simulink model "Quadprog_LF_constraint"  (R2024b)
settings: Solver=FixedStepAuto  StartTime=0.0  StopTime=20  FixedStep=Ts  RelTol=1e-3
model workspace (MAT data in the model file):
  Ts = 0.001
  a = 0.8
settings Model: Creator=sara  LastModifiedBy=Negin Service
settings SolverCC: AlgebraicLoopSolver=TrustRegion
settings RTWCC: GPUComputeCapability=3.5

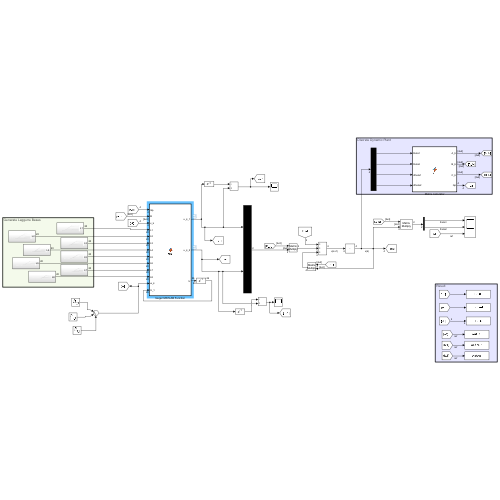
[thumbnail: Simulink's stored preview of the top-level diagram]
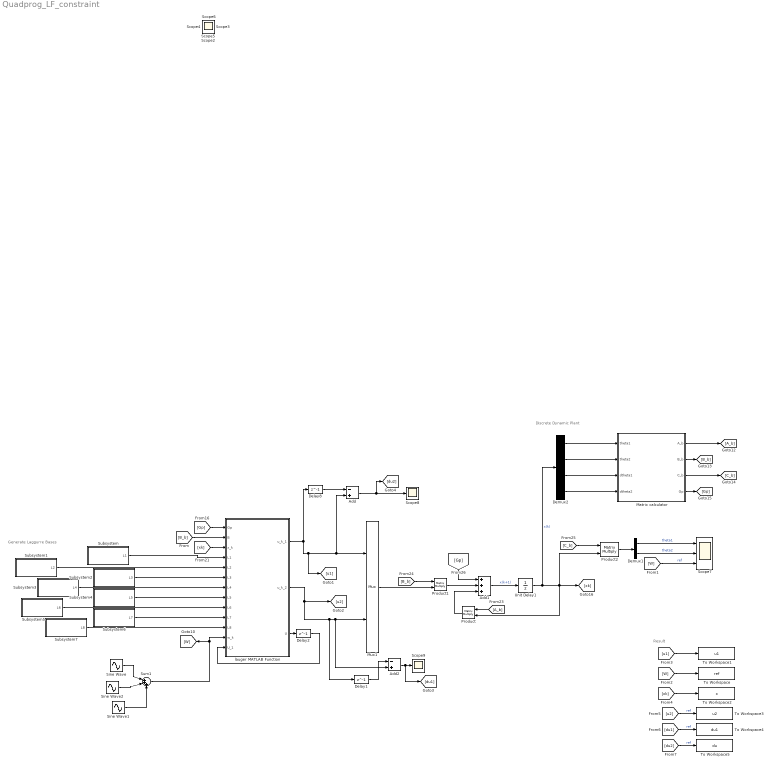
== system Quadprog_LF_constraint ==
  note: Result
  note: Discrete Dynamic Plant
  note: Generate Laggurre Bases
  Add : Sum  Inputs=-+
  Add1 : Sum  Inputs=+++
  Add2 : Sum  Inputs=-+
  Delay1 : Delay  DelayLength=1  SampleTime=Ts
  Delay2 : Delay  DelayLength=1  SampleTime=Ts
  Delay8 : Delay  DelayLength=1  SampleTime=Ts
  Demux1 : Demux  Outputs=2
  Demux2 : Demux
  Matrix calculator : MATLAB Function  TreatAsAtomicUnit=on
  Mux1 : Mux  Inputs=2
  Product : Product  Multiplication=Matrix(*)
  Product1 : Product  Multiplication=Matrix(*)
  Product2 : Product  Multiplication=Matrix(*)
  Scope7 : Scope  NumInputPorts=3
  Scope{,1..6,8..9} (9 alike) : Scope
  Sine Wave : Sin  Amplitude=4  Frequency=0.5  SampleTime=Ts
  Sine Wave1 : Sin  Amplitude=4  SampleTime=Ts
  Sine Wave2 : Sin  Amplitude=4  Frequency=1.5  SampleTime=Ts
  Subsystem : Subsystem
  Subsystem1 : Subsystem
  Subsystem2 : Subsystem
  Subsystem3 : Subsystem
  Subsystem4 : Subsystem
  Subsystem5 : Subsystem
  Subsystem6 : Subsystem
  Subsystem7 : Subsystem
  Sum1 : Sum  Inputs=|+++
  To Workspace : ToWorkspace  VariableName=ref  SaveFormat=Timeseries  SampleTime=-1
  To Workspace1 : ToWorkspace  VariableName=u1  SaveFormat=Timeseries  SampleTime=-1
  To Workspace2 : ToWorkspace  VariableName=x  SaveFormat=Timeseries  SampleTime=-1
  To Workspace3 : ToWorkspace  VariableName=u2  SaveFormat=Timeseries  SampleTime=-1
  To Workspace4 : ToWorkspace  VariableName=du1  SaveFormat=Timeseries  SampleTime=-1
  To Workspace5 : ToWorkspace  VariableName=du  SaveFormat=Timeseries  SampleTime=-1
  Unit Delay1 : UnitDelay  InitialCondition=[0;0;0;0]  SampleTime=Ts  HasFrameUpgradeWarning=on
  lauger MATLAB Function : MATLAB Function  TreatAsAtomicUnit=on
  wires:
  Sine Wave/1 -> Sum1/1
  Subsystem2/1(L3) -> lauger MATLAB Function/6(L3)
  Subsystem/1(L1) -> lauger MATLAB Function/4(L1)
  Subsystem1/1(L2) -> lauger MATLAB Function/5(L2)
  Sum1/1 -> lauger MATLAB Function/12(w_k), [W]
  [B_b] -> lauger MATLAB Function/2(B)
  [xk] -> lauger MATLAB Function/3(x_k)
  [Gp] -> lauger MATLAB Function/1(Gp)
  Mux1/1 -> Product1/2
  Subsystem3/1(L4) -> lauger MATLAB Function/7(L4)
  Subsystem4/1(L5) -> lauger MATLAB Function/8(L5)
  Subsystem5/1(L6) -> lauger MATLAB Function/9(L6)
  Subsystem6/1(L7) -> lauger MATLAB Function/10(L7)
  Subsystem7/1(L8) -> lauger MATLAB Function/11(L8)
  Unit Delay1/1 -> Demux2/1, Product2/2, [xk], Product/2  "x(k)"
  Matrix calculator/1(A_b) -> [A_b]
  Matrix calculator/4(Gp) -> [Gp]
  Matrix calculator/3(C_b) -> [C_b]
  Matrix calculator/2(B_b) -> [B_b]
  [A_b] -> Product/1
  Product/1 -> Add1/3
  [B_b] -> Product1/1
  Product1/1 -> Add1/2
  Add1/1 -> Unit Delay1/1  "x(k+1)"
  [Gp] -> Add1/1
  [C_b] -> Product2/1
  Product2/1 -> Demux1/1
  Demux1/1 -> Scope7/1  "theta1"
  Demux1/2 -> Scope7/2  "theta2"
  Demux2/1 -> Matrix calculator/1(theta1)
  Demux2/2 -> Matrix calculator/2(theta2)
  Demux2/3 -> Matrix calculator/3(dtheta1)
  Demux2/4 -> Matrix calculator/4(dtheta2)
  [W] -> Scope7/3  "ref"
  Sine Wave1/1 -> Sum1/3
  Sine Wave2/1 -> Sum1/2
  Delay8/1 -> Add/1
  Add/1 -> [du2], Scope8/1
  lauger MATLAB Function/1(u_k_1) -> [u1], Add/2, Mux1/1, Delay8/1
  Delay1/1 -> Add2/1
  Add2/1 -> [du1], Scope9/1
  lauger MATLAB Function/2(u_k_2) -> Delay1/1, Add2/2, Mux1/2, [u2]
  [W] -> To Workspace/1
  [u1] -> To Workspace1/1
  [xk] -> To Workspace2/1
  [u2] -> To Workspace3/1  "ref"
  [du1] -> To Workspace4/1  "ref"
  [du2] -> To Workspace5/1  "ref"
  lauger MATLAB Function/3(U) -> Delay2/1
  Delay2/1 -> lauger MATLAB Function/13(U_1)

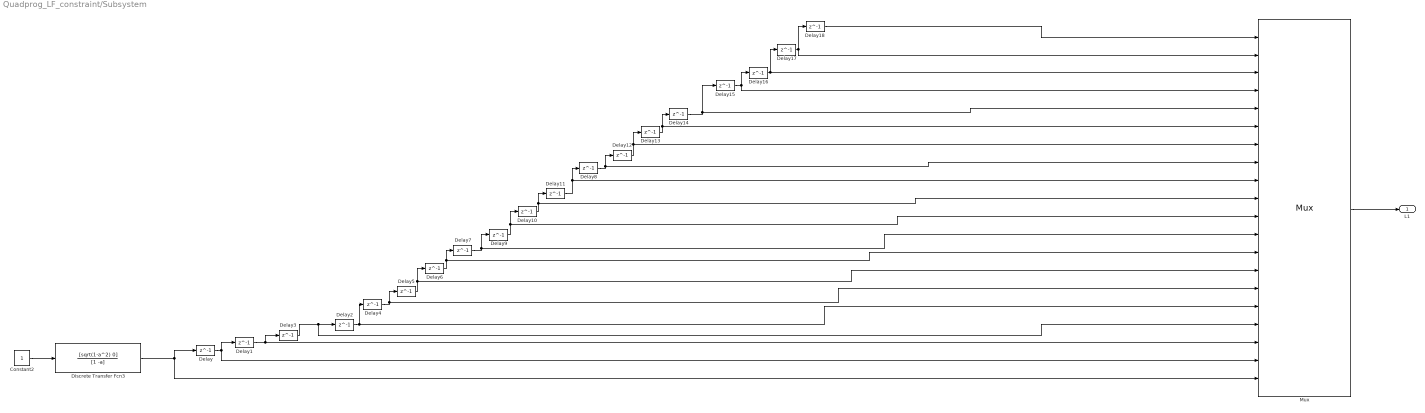
== system Quadprog_LF_constraint/Subsystem ==
  Constant2 : Constant  SampleTime=0.1
  Delay{,1..18} (19 alike) : Delay  DelayLength=1  SampleTime=Ts
  Discrete Transfer Fcn3 : DiscreteTransferFcn  Numerator=[sqrt(1-a^2) 0]  Denominator=[1 -a]  SampleTime=Ts
  Mux : Mux  Inputs=20
  L1 : Outport
  wires:
  Constant2/1 -> Discrete Transfer Fcn3/1
  Delay2/1 -> Mux/16, Delay4/1
  Discrete Transfer Fcn3/1 -> Mux/20, Delay/1
  Delay3/1 -> Mux/17, Delay2/1
  Delay1/1 -> Mux/18, Delay3/1
  Delay/1 -> Mux/19, Delay1/1
  Delay4/1 -> Mux/15, Delay5/1
  Delay5/1 -> Mux/14, Delay6/1
  Delay6/1 -> Mux/13, Delay7/1
  Delay9/1 -> Mux/11, Delay10/1
  Delay7/1 -> Mux/12, Delay9/1
  Delay10/1 -> Mux/10, Delay11/1
  Delay12/1 -> Mux/7, Delay13/1
  Delay8/1 -> Mux/8, Delay12/1
  Delay13/1 -> Delay14/1, Mux/6
  Delay11/1 -> Mux/9, Delay8/1
  Delay16/1 -> Delay17/1, Mux/3
  Delay15/1 -> Delay16/1, Mux/4
  Delay17/1 -> Delay18/1, Mux/2
  Delay14/1 -> Mux/5, Delay15/1
  Mux/1 -> L1/1
  Delay18/1 -> Mux/1

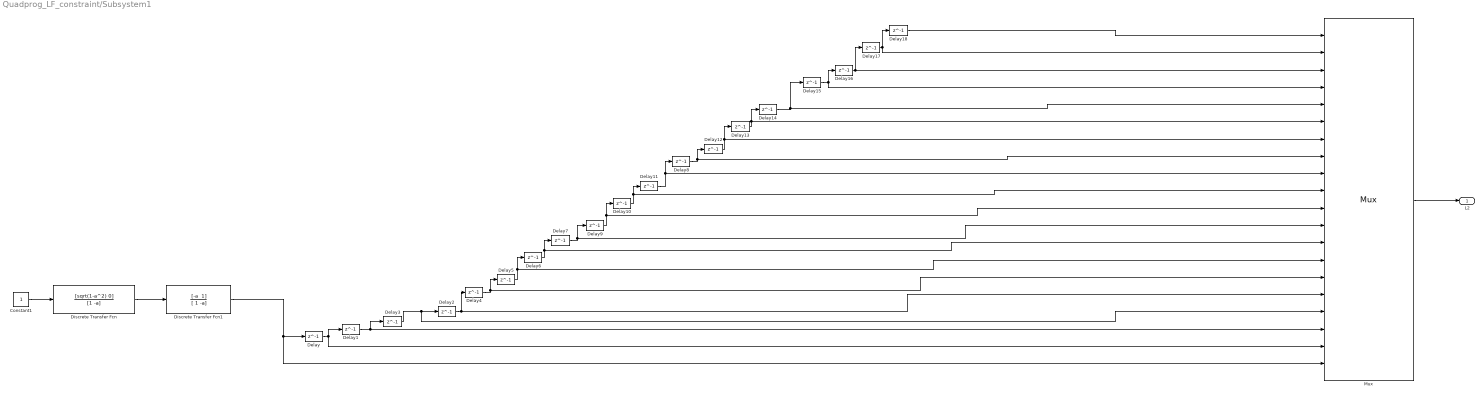
== system Quadprog_LF_constraint/Subsystem1 ==
  Constant1 : Constant  SampleTime=0.1
  Delay{,1..18} (19 alike) : Delay  DelayLength=1  SampleTime=Ts
  Discrete Transfer Fcn : DiscreteTransferFcn  Numerator=[sqrt(1-a^2) 0]  Denominator=[1 -a]  SampleTime=Ts
  Discrete Transfer Fcn1 : DiscreteTransferFcn  Numerator="[-a  1]"  Denominator=[ 1 -a]  SampleTime=Ts
  Mux : Mux  Inputs=20
  L2 : Outport
  wires:
  Delay18/1 -> Mux/1
  Mux/1 -> L2/1
  Delay14/1 -> Delay15/1, Mux/5
  Delay17/1 -> Delay18/1, Mux/2
  Delay15/1 -> Mux/4, Delay16/1
  Delay16/1 -> Mux/3, Delay17/1
  Delay11/1 -> Delay8/1, Mux/9
  Delay13/1 -> Mux/6, Delay14/1
  Delay8/1 -> Delay12/1, Mux/8
  Delay12/1 -> Delay13/1, Mux/7
  Delay10/1 -> Delay11/1, Mux/10
  Delay7/1 -> Delay9/1, Mux/12
  Delay9/1 -> Delay10/1, Mux/11
  Delay6/1 -> Delay7/1, Mux/13
  Delay5/1 -> Delay6/1, Mux/14
  Delay4/1 -> Delay5/1, Mux/15
  Delay/1 -> Delay1/1, Mux/19
  Delay1/1 -> Delay3/1, Mux/18
  Delay3/1 -> Delay2/1, Mux/17
  Discrete Transfer Fcn1/1 -> Mux/20, Delay/1
  Delay2/1 -> Delay4/1, Mux/16
  Discrete Transfer Fcn/1 -> Discrete Transfer Fcn1/1
  Constant1/1 -> Discrete Transfer Fcn/1

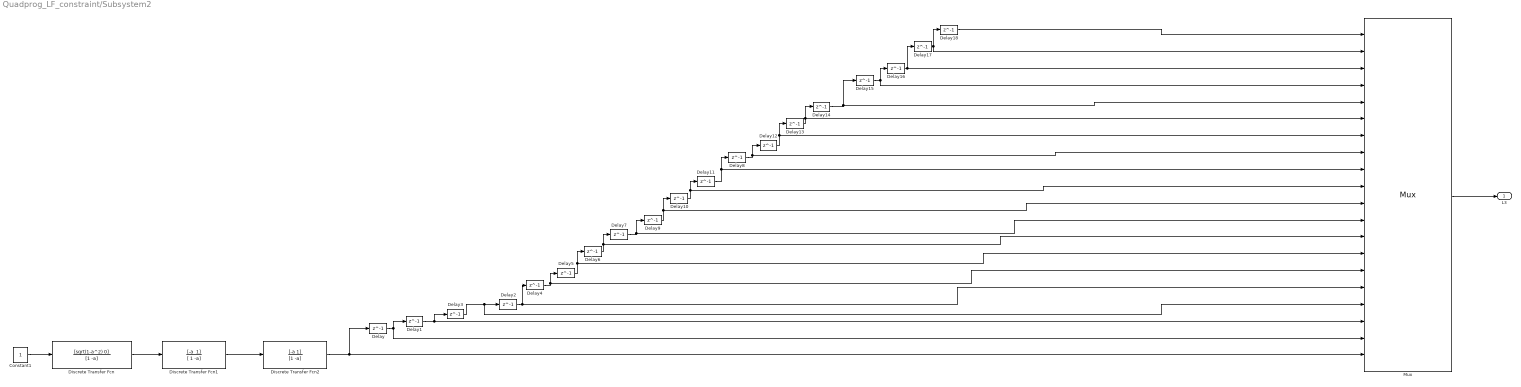
== system Quadprog_LF_constraint/Subsystem2 ==
  Constant1 : Constant  SampleTime=0.1
  Delay{,1..18} (19 alike) : Delay  DelayLength=1  SampleTime=Ts
  Discrete Transfer Fcn : DiscreteTransferFcn  Numerator=[sqrt(1-a^2) 0]  Denominator=[1 -a]  SampleTime=Ts
  Discrete Transfer Fcn1 : DiscreteTransferFcn  Numerator="[-a  1]"  Denominator=[ 1 -a]  SampleTime=Ts
  Discrete Transfer Fcn2 : DiscreteTransferFcn  Numerator=[-a 1]  Denominator=[1 -a]  SampleTime=Ts
  Mux : Mux  Inputs=20
  L3 : Outport
  wires:
  Delay2/1 -> Mux/16, Delay4/1
  Discrete Transfer Fcn2/1 -> Delay/1, Mux/20
  Delay3/1 -> Mux/17, Delay2/1
  Delay1/1 -> Mux/18, Delay3/1
  Delay/1 -> Mux/19, Delay1/1
  Delay4/1 -> Mux/15, Delay5/1
  Delay5/1 -> Mux/14, Delay6/1
  Delay6/1 -> Mux/13, Delay7/1
  Delay9/1 -> Mux/11, Delay10/1
  Delay7/1 -> Mux/12, Delay9/1
  Delay10/1 -> Mux/10, Delay11/1
  Delay12/1 -> Mux/7, Delay13/1
  Delay8/1 -> Mux/8, Delay12/1
  Delay13/1 -> Delay14/1, Mux/6
  Delay11/1 -> Mux/9, Delay8/1
  Delay16/1 -> Delay17/1, Mux/3
  Delay15/1 -> Delay16/1, Mux/4
  Delay17/1 -> Delay18/1, Mux/2
  Delay14/1 -> Mux/5, Delay15/1
  Mux/1 -> L3/1
  Delay18/1 -> Mux/1
  Discrete Transfer Fcn/1 -> Discrete Transfer Fcn1/1
  Discrete Transfer Fcn1/1 -> Discrete Transfer Fcn2/1
  Constant1/1 -> Discrete Transfer Fcn/1

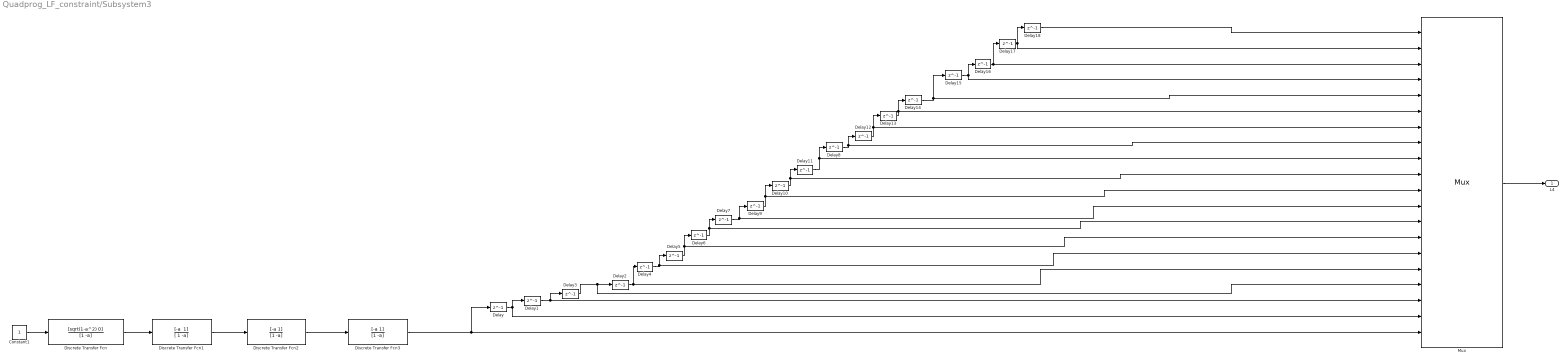
== system Quadprog_LF_constraint/Subsystem3 ==
  Constant1 : Constant  SampleTime=0.1
  Delay{,1..18} (19 alike) : Delay  DelayLength=1  SampleTime=Ts
  Discrete Transfer Fcn : DiscreteTransferFcn  Numerator=[sqrt(1-a^2) 0]  Denominator=[1 -a]  SampleTime=Ts
  Discrete Transfer Fcn1 : DiscreteTransferFcn  Numerator="[-a  1]"  Denominator=[ 1 -a]  SampleTime=Ts
  Discrete Transfer Fcn2 : DiscreteTransferFcn  Numerator=[-a 1]  Denominator=[1 -a]  SampleTime=Ts
  Discrete Transfer Fcn3 : DiscreteTransferFcn  Numerator=[-a 1]  Denominator=[1 -a]  SampleTime=Ts
  Mux : Mux  Inputs=20
  L4 : Outport
  wires:
  Constant1/1 -> Discrete Transfer Fcn/1
  Discrete Transfer Fcn1/1 -> Discrete Transfer Fcn2/1
  Discrete Transfer Fcn/1 -> Discrete Transfer Fcn1/1
  Delay18/1 -> Mux/1
  Mux/1 -> L4/1
  Delay14/1 -> Delay15/1, Mux/5
  Delay17/1 -> Mux/2, Delay18/1
  Delay15/1 -> Mux/4, Delay16/1
  Delay16/1 -> Mux/3, Delay17/1
  Delay11/1 -> Delay8/1, Mux/9
  Delay13/1 -> Mux/6, Delay14/1
  Delay8/1 -> Delay12/1, Mux/8
  Delay12/1 -> Delay13/1, Mux/7
  Delay10/1 -> Delay11/1, Mux/10
  Delay7/1 -> Delay9/1, Mux/12
  Delay9/1 -> Delay10/1, Mux/11
  Delay6/1 -> Delay7/1, Mux/13
  Delay5/1 -> Delay6/1, Mux/14
  Delay4/1 -> Delay5/1, Mux/15
  Delay/1 -> Delay1/1, Mux/19
  Delay1/1 -> Delay3/1, Mux/18
  Delay3/1 -> Delay2/1, Mux/17
  Discrete Transfer Fcn3/1 -> Mux/20, Delay/1
  Delay2/1 -> Delay4/1, Mux/16
  Discrete Transfer Fcn2/1 -> Discrete Transfer Fcn3/1

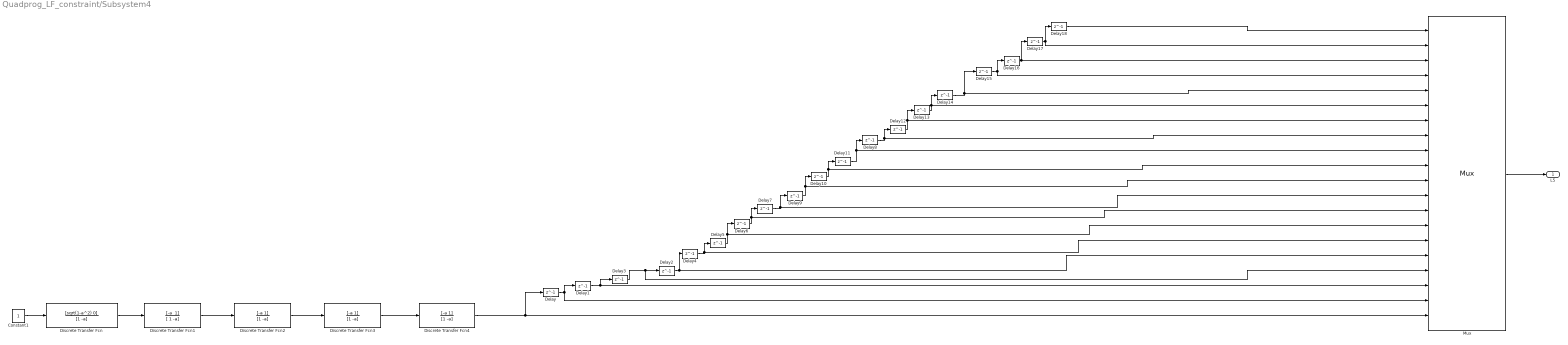
== system Quadprog_LF_constraint/Subsystem4 ==
  Constant1 : Constant  SampleTime=0.1
  Delay{,1..18} (19 alike) : Delay  DelayLength=1  SampleTime=Ts
  Discrete Transfer Fcn : DiscreteTransferFcn  Numerator=[sqrt(1-a^2) 0]  Denominator=[1 -a]  SampleTime=Ts
  Discrete Transfer Fcn1 : DiscreteTransferFcn  Numerator="[-a  1]"  Denominator=[ 1 -a]  SampleTime=Ts
  Discrete Transfer Fcn2 : DiscreteTransferFcn  Numerator=[-a 1]  Denominator=[1 -a]  SampleTime=Ts
  Discrete Transfer Fcn3 : DiscreteTransferFcn  Numerator=[-a 1]  Denominator=[1 -a]  SampleTime=Ts
  Discrete Transfer Fcn4 : DiscreteTransferFcn  Numerator=[-a 1]  Denominator=[1 -a]  SampleTime=Ts
  Mux : Mux  Inputs=20
  L5 : Outport
  wires:
  Delay2/1 -> Mux/16, Delay4/1
  Discrete Transfer Fcn2/1 -> Discrete Transfer Fcn3/1
  Delay3/1 -> Mux/17, Delay2/1
  Delay1/1 -> Mux/18, Delay3/1
  Delay/1 -> Mux/19, Delay1/1
  Delay4/1 -> Mux/15, Delay5/1
  Delay5/1 -> Mux/14, Delay6/1
  Delay6/1 -> Mux/13, Delay7/1
  Delay9/1 -> Mux/11, Delay10/1
  Delay7/1 -> Mux/12, Delay9/1
  Delay10/1 -> Mux/10, Delay11/1
  Delay12/1 -> Mux/7, Delay13/1
  Delay8/1 -> Mux/8, Delay12/1
  Delay13/1 -> Delay14/1, Mux/6
  Delay11/1 -> Mux/9, Delay8/1
  Delay16/1 -> Delay17/1, Mux/3
  Delay15/1 -> Delay16/1, Mux/4
  Delay17/1 -> Delay18/1, Mux/2
  Delay14/1 -> Mux/5, Delay15/1
  Mux/1 -> L5/1
  Delay18/1 -> Mux/1
  Discrete Transfer Fcn/1 -> Discrete Transfer Fcn1/1
  Discrete Transfer Fcn1/1 -> Discrete Transfer Fcn2/1
  Constant1/1 -> Discrete Transfer Fcn/1
  Discrete Transfer Fcn3/1 -> Discrete Transfer Fcn4/1
  Discrete Transfer Fcn4/1 -> Delay/1, Mux/20

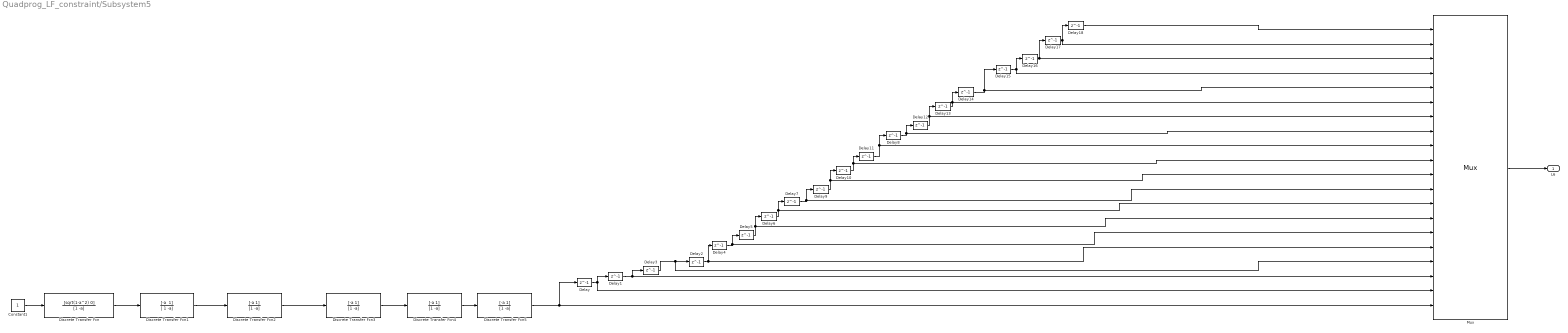
== system Quadprog_LF_constraint/Subsystem5 ==
  Constant1 : Constant  SampleTime=0.1
  Delay{,1..18} (19 alike) : Delay  DelayLength=1  SampleTime=Ts
  Discrete Transfer Fcn : DiscreteTransferFcn  Numerator=[sqrt(1-a^2) 0]  Denominator=[1 -a]  SampleTime=Ts
  Discrete Transfer Fcn1 : DiscreteTransferFcn  Numerator="[-a  1]"  Denominator=[ 1 -a]  SampleTime=Ts
  Discrete Transfer Fcn{2..5} (4 alike) : DiscreteTransferFcn  Numerator=[-a 1]  Denominator=[1 -a]  SampleTime=Ts
  Mux : Mux  Inputs=20
  L6 : Outport
  wires:
  Constant1/1 -> Discrete Transfer Fcn/1
  Discrete Transfer Fcn1/1 -> Discrete Transfer Fcn2/1
  Discrete Transfer Fcn/1 -> Discrete Transfer Fcn1/1
  Delay18/1 -> Mux/1
  Mux/1 -> L6/1
  Delay14/1 -> Delay15/1, Mux/5
  Delay17/1 -> Mux/2, Delay18/1
  Delay15/1 -> Mux/4, Delay16/1
  Delay16/1 -> Mux/3, Delay17/1
  Delay11/1 -> Delay8/1, Mux/9
  Delay13/1 -> Mux/6, Delay14/1
  Delay8/1 -> Delay12/1, Mux/8
  Delay12/1 -> Delay13/1, Mux/7
  Delay10/1 -> Delay11/1, Mux/10
  Delay7/1 -> Delay9/1, Mux/12
  Delay9/1 -> Delay10/1, Mux/11
  Delay6/1 -> Delay7/1, Mux/13
  Delay5/1 -> Delay6/1, Mux/14
  Delay4/1 -> Delay5/1, Mux/15
  Delay/1 -> Delay1/1, Mux/19
  Delay1/1 -> Delay3/1, Mux/18
  Delay3/1 -> Delay2/1, Mux/17
  Discrete Transfer Fcn2/1 -> Discrete Transfer Fcn3/1
  Delay2/1 -> Delay4/1, Mux/16
  Discrete Transfer Fcn3/1 -> Discrete Transfer Fcn4/1
  Discrete Transfer Fcn4/1 -> Discrete Transfer Fcn5/1
  Discrete Transfer Fcn5/1 -> Mux/20, Delay/1

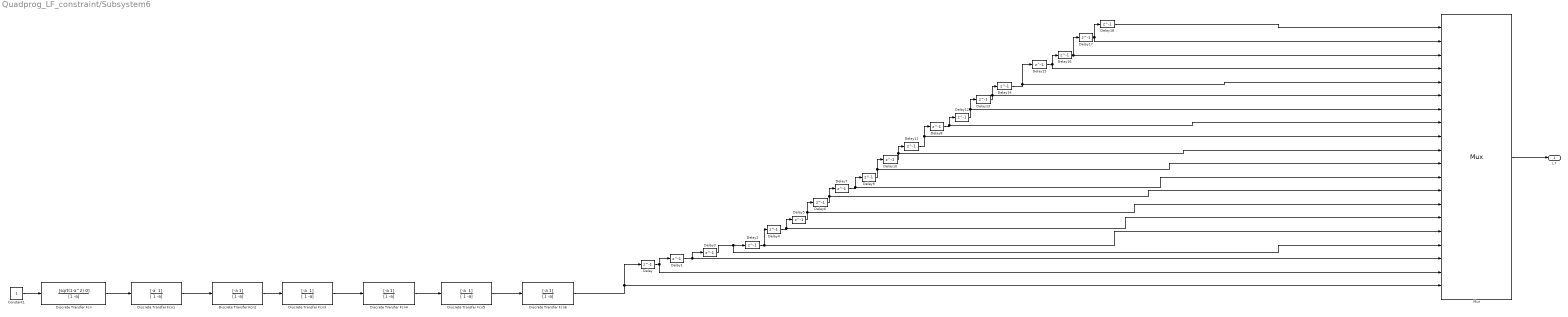
== system Quadprog_LF_constraint/Subsystem6 ==
  Constant1 : Constant  SampleTime=0.1
  Delay{,1..18} (19 alike) : Delay  DelayLength=1  SampleTime=Ts
  Discrete Transfer Fcn : DiscreteTransferFcn  Numerator=[sqrt(1-a^2) 0]  Denominator=[1 -a]  SampleTime=Ts
  Discrete Transfer Fcn1 : DiscreteTransferFcn  Numerator="[-a  1]"  Denominator=[ 1 -a]  SampleTime=Ts
  Discrete Transfer Fcn2 : DiscreteTransferFcn  Numerator=[-a 1]  Denominator=[1 -a]  SampleTime=Ts
  Discrete Transfer Fcn3 : DiscreteTransferFcn  Numerator="[-a  1]"  Denominator=[ 1 -a]  SampleTime=Ts
  Discrete Transfer Fcn4 : DiscreteTransferFcn  Numerator=[-a 1]  Denominator=[1 -a]  SampleTime=Ts
  Discrete Transfer Fcn5 : DiscreteTransferFcn  Numerator="[-a  1]"  Denominator=[ 1 -a]  SampleTime=Ts
  Discrete Transfer Fcn6 : DiscreteTransferFcn  Numerator=[-a 1]  Denominator=[1 -a]  SampleTime=Ts
  Mux : Mux  Inputs=20
  L7 : Outport
  wires:
  Delay2/1 -> Mux/16, Delay4/1
  Discrete Transfer Fcn6/1 -> Delay/1, Mux/20
  Delay3/1 -> Mux/17, Delay2/1
  Delay1/1 -> Mux/18, Delay3/1
  Delay/1 -> Mux/19, Delay1/1
  Delay4/1 -> Mux/15, Delay5/1
  Delay5/1 -> Mux/14, Delay6/1
  Delay6/1 -> Mux/13, Delay7/1
  Delay9/1 -> Mux/11, Delay10/1
  Delay7/1 -> Mux/12, Delay9/1
  Delay10/1 -> Mux/10, Delay11/1
  Delay12/1 -> Mux/7, Delay13/1
  Delay8/1 -> Mux/8, Delay12/1
  Delay13/1 -> Delay14/1, Mux/6
  Delay11/1 -> Mux/9, Delay8/1
  Delay16/1 -> Delay17/1, Mux/3
  Delay15/1 -> Delay16/1, Mux/4
  Delay17/1 -> Delay18/1, Mux/2
  Delay14/1 -> Mux/5, Delay15/1
  Mux/1 -> L7/1
  Delay18/1 -> Mux/1
  Discrete Transfer Fcn/1 -> Discrete Transfer Fcn1/1
  Discrete Transfer Fcn1/1 -> Discrete Transfer Fcn2/1
  Constant1/1 -> Discrete Transfer Fcn/1
  Discrete Transfer Fcn3/1 -> Discrete Transfer Fcn4/1
  Discrete Transfer Fcn2/1 -> Discrete Transfer Fcn3/1
  Discrete Transfer Fcn5/1 -> Discrete Transfer Fcn6/1
  Discrete Transfer Fcn4/1 -> Discrete Transfer Fcn5/1

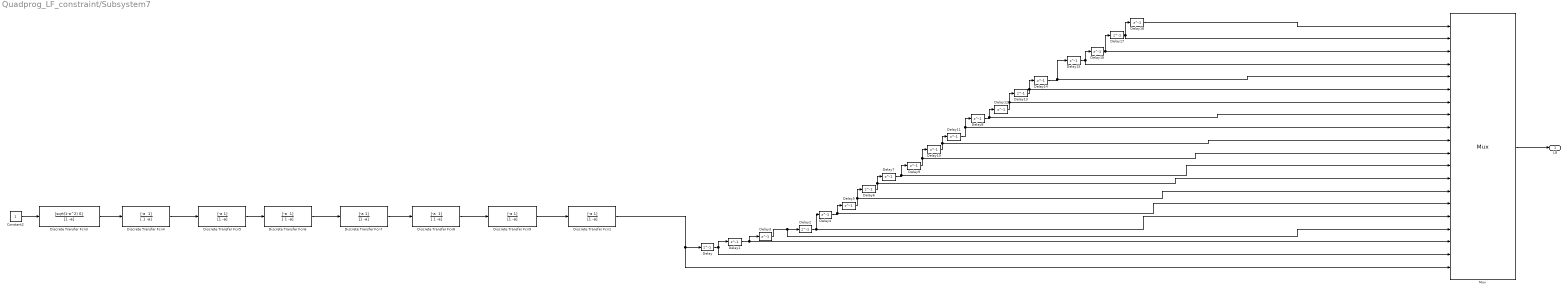
== system Quadprog_LF_constraint/Subsystem7 ==
  Constant2 : Constant  SampleTime=0.1
  Delay{,1..18} (19 alike) : Delay  DelayLength=1  SampleTime=Ts
  Discrete Transfer Fcn{1,5,7,9} (4 alike) : DiscreteTransferFcn  Numerator=[-a 1]  Denominator=[1 -a]  SampleTime=Ts
  Discrete Transfer Fcn3 : DiscreteTransferFcn  Numerator=[sqrt(1-a^2) 0]  Denominator=[1 -a]  SampleTime=Ts
  Discrete Transfer Fcn4 : DiscreteTransferFcn  Numerator="[-a  1]"  Denominator=[ 1 -a]  SampleTime=Ts
  Discrete Transfer Fcn6 : DiscreteTransferFcn  Numerator="[-a  1]"  Denominator=[ 1 -a]  SampleTime=Ts
  Discrete Transfer Fcn8 : DiscreteTransferFcn  Numerator="[-a  1]"  Denominator=[ 1 -a]  SampleTime=Ts
  Mux : Mux  Inputs=20
  L8 : Outport
  wires:
  Delay18/1 -> Mux/1
  Mux/1 -> L8/1
  Delay14/1 -> Delay15/1, Mux/5
  Delay17/1 -> Mux/2, Delay18/1
  Delay15/1 -> Mux/4, Delay16/1
  Delay16/1 -> Mux/3, Delay17/1
  Delay11/1 -> Delay8/1, Mux/9
  Delay13/1 -> Mux/6, Delay14/1
  Delay8/1 -> Delay12/1, Mux/8
  Delay12/1 -> Delay13/1, Mux/7
  Delay10/1 -> Delay11/1, Mux/10
  Delay7/1 -> Delay9/1, Mux/12
  Delay9/1 -> Delay10/1, Mux/11
  Delay6/1 -> Delay7/1, Mux/13
  Delay5/1 -> Delay6/1, Mux/14
  Delay4/1 -> Delay5/1, Mux/15
  Delay/1 -> Delay1/1, Mux/19
  Delay1/1 -> Delay3/1, Mux/18
  Delay3/1 -> Delay2/1, Mux/17
  Discrete Transfer Fcn1/1 -> Mux/20, Delay/1
  Delay2/1 -> Delay4/1, Mux/16
  Discrete Transfer Fcn5/1 -> Discrete Transfer Fcn6/1
  Constant2/1 -> Discrete Transfer Fcn3/1
  Discrete Transfer Fcn4/1 -> Discrete Transfer Fcn5/1
  Discrete Transfer Fcn6/1 -> Discrete Transfer Fcn7/1
  Discrete Transfer Fcn3/1 -> Discrete Transfer Fcn4/1
  Discrete Transfer Fcn7/1 -> Discrete Transfer Fcn8/1
  Discrete Transfer Fcn8/1 -> Discrete Transfer Fcn9/1
  Discrete Transfer Fcn9/1 -> Discrete Transfer Fcn1/1

== matlab function Quadprog_LF_constraint/lauger MATLAB Function ==
  data: Gp input; B input; x_k input; L1 input; u_k_1 output; L2 input; L3 input; L4 input; L5 input; L6 input; L7 input; L8 input; w_k input; U_1 input; u_k_2 output; Ts parameter; U output
function [u_k_1,u_k_2,U] = fcn(Gp,B,x_k,L1,L2,L3,L4,L5,L6,L7,L8,w_k,U_1, Ts)
    T  = Ts;
    A  = [eye(2) , T*eye(2); zeros(2), eye(2)];
    C  = [1 0 0 0 ;0 1 0 0];
    
    Np = 15;
    m  = 15;
    r  = 8;
    %%%%%%%%%%%    adjustable parameters
    Q  = 500*eye(2*Np);
    RL = 500*eye(2*r);
    
    %%%%%%%%%%%   calculating matrix W , F , F_2
    W   =  zeros(2*Np,1);
    F   =  zeros(2*Np,4);
    F_2 =  zeros(2*Np,4);
    for i=1:2*Np
        W(i) = w_k;
    end
    for i=1:Np
        
        F(2*i-1:2*i,:)  =  C*A^i;
        if i == 1
            F_2(1:2,:)=C;
        else
            F_2(2*i-1:2*i,:) = C*A^(i-1) + F_2(2*(i-1)-1:2*(i-1),:);
        end
    end
    
    
    %%%%%%%%%%%   calculate matrix L
    L1       =  L1(1:m);   % L1 = [l1(k) l1(k+1) l1(k+2) . . .  l1(k+m-1)]'
    L2       =  L2(1:m);
    L3       =  L3(1:m);
    L4       =  L4(1:m);   
    L5       =  L5(1:m);
    L6       =  L6(1:m);
    L7       =  L7(1:m);   
    L8       =  L8(1:m);
    
    L_temp   =  zeros(1,m);       % temporary parameter
    L        =  zeros(2*r,2*m);   % main L matrix that we want to calc
    for i = 1:r
        if i == 1
            L_temp = L1;
        elseif i==2
            L_temp = L2;
        elseif i==3
            L_temp = L3;
        elseif i==4
            L_temp = L4;
        elseif i==5
            L_temp = L5;
        elseif i==6
            L_temp = L6;
        elseif i==7
            L_temp = L7;
        elseif i==8
            L_temp = L8;
        end
        row      =  zeros(1,2*m);  % temporary parameter
        for j = 1:(2*m)
            if mod(j,2) ~= 0
                row(1,j) = L_temp((j+1)/2);
            end
            L(i,:)=row;
            L(i+r,2:end)=row(1,1:(end-1));
        end
        
    end
    
    %%%%%%%%%%%  calculate matrix Phi
    col =zeros(2*Np,2);   %% dimension = 10*2
    
    for i=1:Np
        col((2*i-1):(2*i),:)=C*A^(i-1)*B;
    end
    
    Phi=zeros(2*Np,2*m);
    
    for i=0:(m-1)
        col2=[zeros(2*i,2);col(1:end-(2*i),:)];
        Phi(:,(i+1)*2-1:(i+1)*2)=col2;
    end
    
    
    
    
    
    %%   quad calculataions
    f    =   2* L  * Phi' * Q *( F*x_k  + F_2*Gp -  W );
    H    =   2*(L*Phi'*Q*Phi*L'+RL);
    coder.extrinsic('quadprog')
    
    

%     
%     %%%%%%%%%%%  calculate matrix Phi_quad
%     col_quad  = zeros(4*Np,2);   %% 
%     
%     for i=1:Np
%         col_quad((4*i-3):(4*i),:)=A^(i-1)*B;
%     end
%     
%     Phi_quad  = zeros(4*Np,2*m);
%     
%     for i=0:(m-1)
%         col2_quad  =   [zeros(4*i,2);col_quad(1:end-(4*i),:)];
%         Phi_quad(:,(i+1)*2-1:(i+1)*2)  =   col2_quad;
%     end 
    
    
    
    
    
    
    
    
    
    eta  =   zeros(2*r,1);
    

    b = zeros(8*m,1);
    for i=1:4*m
        b(i)=2;
    end
    
    for i = (4*m+1):8*m
        b(i)=0.25;
    end
    b(4*m+1:6*m,1)  =  b(4*m+1:6*m,1)  +  U_1  ;
    b(6*m+1:8*m,1)  =  b(6*m+1:8*m,1)  -  U_1  ;
    
    
    A=[  L'  ;  -L' ;  L'   ; - L'];
    eta  = quadprog(H,f,A,b);
    
    
    
    
    U            =  L'*eta;
    u_k_1        =  U(1);
    u_k_2        =  U(2);
    
    
end

== matlab function Quadprog_LF_constraint/Matrix calculator ==
  data: theta1 input; A_b output; theta2 input; dtheta1 input; dtheta2 input; B_b output; C_b output; Gp output; Ts parameter
function [A_b,B_b,C_b,Gp]= fcn(theta1,theta2,dtheta1,dtheta2, Ts)
T  = Ts;
m1 = 0.67;
m2 = 0.33;
l1 = 0.18;
l2 = 0.07;
r1 = l1/2; %?
r2 = l2/2;  %?
g  = 9.8;
I1 = (1/12)*m1*l1^2;
I2 = (1/12)*m2*l2^2;

% Precomputing trigonometric terms


c1  = cos(theta1);
s1  = sin(theta1);
c2  = cos(theta2);
s2  = sin(theta2);
c12 = cos(theta1 + theta2);
s12 = sin(theta1 + theta2);


x = [theta1 ; theta2; dtheta1 ; dtheta2];
% Mass matrix M(q)
M11 = m1*r1^2 + m2*(l1^2 + r2^2 + 2*l1*r2*c2) + I1 + I2;
M12 = m2*(r2^2 + l1*r2*c2) + I2;
M21 = M12;
M22 = m2*r2^2 + I2;
M   = [M11, M12; M21, M22];

% Coriolis and centripetal matrix C(q, q_dot)
C11 = -m2*l1*r2*s2*dtheta2;
C12 = -m2*l1*r2*s2*(dtheta1 + dtheta2);
C21 = m2*l1*r2*s2*dtheta1;
C22 = 0;
C   = [C11, C12; C21, C22];

% Gravity vector G(q)
G1 = (m1*r2 + m2*l1)*g*c1 + m2*r2*g*c12;
G2 = m2*r2*g*c12;
G  = [G1; G2];
P2 = inv(M);
P1 = eye(2);


f1 = 0;
f2 = -inv(M)*(C*x(3:4)+G);


%  x_b(k+1) = A_b*x_b(k) + B_b*u_b(k)  + Gp   (eq4 in article)
%  y_b(k)   = C_b*x_b(k)
A_b   = [eye(2) , T*eye(2); zeros(2), eye(2)];
B_b   = [(T^2/2)*(P2); T*P2];

Gp    = [(T^2/2)*f2; T*f2];
C_b   = [eye(2) zeros(2)];
